simulink model "FKtest"  (Simulink 6.6)
settings: Solver=ode4  StartTime=0.0  StopTime=400  FixedStep=0.05  RelTol=1e-3
undefined symbols (not defined in the file or in its folder): amp2, vessel
libraries: marine_gnc x21, simulink x5
(part 3 of 3)

== system FKtest/Wave loads for heading2/Wave component loop/Force RAO tables/RAO interpolation in frequency5 ==
  Table : Inport
  omega : Inport  Port=2
  beta_idx : Inport  Port=3
  U_idx : Inport  Port=4
  Demux : Demux  Outputs=2
  Mux : Mux  Inputs=2
  Prelookup1 : PreLookup  BreakpointsData=vessel.forceRAO.w  BeginIndexSearchUsingPreviousIndexResult=on  ProcessOutOfRangeInput=Linear extrapolation
  Product : Product  RndMeth=Zero
  Selector1 : Selector  NumberOfDimensions=3  IndexOptions=Index vector (port),Index vector (port),Index vector (port)  Indices=[1 3],1,1  OutputSizes=1,1,1
  Sum1 : Sum  Inputs=++|
  Sum2 : Sum  Inputs=++|
  Sum3 : Sum  Inputs=-+|
  Sum4 : Sum  Inputs=++|
  one : Constant
  y : Outport
  wires:
  Prelookup1/1 -> Sum2/1
  Table/1 -> Selector1/1
  beta_idx/1 -> Selector1/3
  omega/1 -> Prelookup1/1
  U_idx/1 -> Selector1/4
  Sum4/1 -> y/1
  Sum3/1 -> Product/1
  Product/1 -> Sum4/2
  Demux/1 -> Sum4/1, Sum3/1  "y1"
  Demux/2 -> Sum3/2  "y2"
  Prelookup1/2 -> Product/2  "k"
  Selector1/1 -> Demux/1  "y"
  one/1 -> Sum1/2, Sum2/2
  Sum1/1 -> Mux/2
  Sum2/1 -> Sum1/1, Mux/1
  Mux/1 -> Selector1/2

== system FKtest/Wave loads for heading2/Wave component loop/Force RAO tables/RAO interpolation in frequency6 ==
  Table : Inport
  omega : Inport  Port=2
  beta_idx : Inport  Port=3
  U_idx : Inport  Port=4
  Demux : Demux  Outputs=2
  Mux : Mux  Inputs=2
  Prelookup1 : PreLookup  BreakpointsData=vessel.forceRAO.w  BeginIndexSearchUsingPreviousIndexResult=on  ProcessOutOfRangeInput=Linear extrapolation
  Product : Product  RndMeth=Zero
  Selector1 : Selector  NumberOfDimensions=3  IndexOptions=Index vector (port),Index vector (port),Index vector (port)  Indices=[1 3],1,1  OutputSizes=1,1,1
  Sum1 : Sum  Inputs=++|
  Sum2 : Sum  Inputs=++|
  Sum3 : Sum  Inputs=-+|
  Sum4 : Sum  Inputs=++|
  one : Constant
  y : Outport
  wires:
  Prelookup1/1 -> Sum2/1
  Table/1 -> Selector1/1
  beta_idx/1 -> Selector1/3
  omega/1 -> Prelookup1/1
  U_idx/1 -> Selector1/4
  Sum4/1 -> y/1
  Sum3/1 -> Product/1
  Product/1 -> Sum4/2
  Demux/1 -> Sum4/1, Sum3/1  "y1"
  Demux/2 -> Sum3/2  "y2"
  Prelookup1/2 -> Product/2  "k"
  Selector1/1 -> Demux/1  "y"
  one/1 -> Sum1/2, Sum2/2
  Sum1/1 -> Mux/2
  Sum2/1 -> Sum1/1, Mux/1
  Mux/1 -> Selector1/2

== system FKtest/Wave loads for heading2/Wave component loop/Force RAO tables/RAO interpolation in frequency7 ==
  Table : Inport
  omega : Inport  Port=2
  beta_idx : Inport  Port=3
  U_idx : Inport  Port=4
  Demux : Demux  Outputs=2
  Mux : Mux  Inputs=2
  Prelookup1 : PreLookup  BreakpointsData=vessel.forceRAO.w  BeginIndexSearchUsingPreviousIndexResult=on  ProcessOutOfRangeInput=Linear extrapolation
  Product : Product  RndMeth=Zero
  Selector1 : Selector  NumberOfDimensions=3  IndexOptions=Index vector (port),Index vector (port),Index vector (port)  Indices=[1 3],1,1  OutputSizes=1,1,1
  Sum1 : Sum  Inputs=++|
  Sum2 : Sum  Inputs=++|
  Sum3 : Sum  Inputs=-+|
  Sum4 : Sum  Inputs=++|
  one : Constant
  y : Outport
  wires:
  Prelookup1/1 -> Sum2/1
  Table/1 -> Selector1/1
  beta_idx/1 -> Selector1/3
  omega/1 -> Prelookup1/1
  U_idx/1 -> Selector1/4
  Sum4/1 -> y/1
  Sum3/1 -> Product/1
  Product/1 -> Sum4/2
  Demux/1 -> Sum4/1, Sum3/1  "y1"
  Demux/2 -> Sum3/2  "y2"
  Prelookup1/2 -> Product/2  "k"
  Selector1/1 -> Demux/1  "y"
  one/1 -> Sum1/2, Sum2/2
  Sum1/1 -> Mux/2
  Sum2/1 -> Sum1/1, Mux/1
  Mux/1 -> Selector1/2

== system FKtest/Wave loads for heading2/Wave component loop/Force RAO tables/RAO interpolation in frequency8 ==
  Table : Inport
  omega : Inport  Port=2
  beta_idx : Inport  Port=3
  U_idx : Inport  Port=4
  Demux : Demux  Outputs=2
  Mux : Mux  Inputs=2
  Prelookup1 : PreLookup  BreakpointsData=vessel.forceRAO.w  BeginIndexSearchUsingPreviousIndexResult=on  ProcessOutOfRangeInput=Linear extrapolation
  Product : Product  RndMeth=Zero
  Selector1 : Selector  NumberOfDimensions=3  IndexOptions=Index vector (port),Index vector (port),Index vector (port)  Indices=[1 3],1,1  OutputSizes=1,1,1
  Sum1 : Sum  Inputs=++|
  Sum2 : Sum  Inputs=++|
  Sum3 : Sum  Inputs=-+|
  Sum4 : Sum  Inputs=++|
  one : Constant
  y : Outport
  wires:
  Prelookup1/1 -> Sum2/1
  Table/1 -> Selector1/1
  beta_idx/1 -> Selector1/3
  omega/1 -> Prelookup1/1
  U_idx/1 -> Selector1/4
  Sum4/1 -> y/1
  Sum3/1 -> Product/1
  Product/1 -> Sum4/2
  Demux/1 -> Sum4/1, Sum3/1  "y1"
  Demux/2 -> Sum3/2  "y2"
  Prelookup1/2 -> Product/2  "k"
  Selector1/1 -> Demux/1  "y"
  one/1 -> Sum1/2, Sum2/2
  Sum1/1 -> Mux/2
  Sum2/1 -> Sum1/1, Mux/1
  Mux/1 -> Selector1/2

== system FKtest/Wave loads for heading2/Wave component loop/Force RAO tables/RAO interpolation in frequency9 ==
  Table : Inport
  omega : Inport  Port=2
  beta_idx : Inport  Port=3
  U_idx : Inport  Port=4
  Demux : Demux  Outputs=2
  Mux : Mux  Inputs=2
  Prelookup1 : PreLookup  BreakpointsData=vessel.forceRAO.w  BeginIndexSearchUsingPreviousIndexResult=on  ProcessOutOfRangeInput=Linear extrapolation
  Product : Product  RndMeth=Zero
  Selector1 : Selector  NumberOfDimensions=3  IndexOptions=Index vector (port),Index vector (port),Index vector (port)  Indices=[1 3],1,1  OutputSizes=1,1,1
  Sum1 : Sum  Inputs=++|
  Sum2 : Sum  Inputs=++|
  Sum3 : Sum  Inputs=-+|
  Sum4 : Sum  Inputs=++|
  one : Constant
  y : Outport
  wires:
  Prelookup1/1 -> Sum2/1
  Table/1 -> Selector1/1
  beta_idx/1 -> Selector1/3
  omega/1 -> Prelookup1/1
  U_idx/1 -> Selector1/4
  Sum4/1 -> y/1
  Sum3/1 -> Product/1
  Product/1 -> Sum4/2
  Demux/1 -> Sum4/1, Sum3/1  "y1"
  Demux/2 -> Sum3/2  "y2"
  Prelookup1/2 -> Product/2  "k"
  Selector1/1 -> Demux/1  "y"
  one/1 -> Sum1/2, Sum2/2
  Sum1/1 -> Mux/2
  Sum2/1 -> Sum1/1, Mux/1
  Mux/1 -> Selector1/2

== system FKtest/Wave loads for heading2/Wave component loop/WD RAO tables/RAO interpolation in frequency1 ==
  Table : Inport
  omega : Inport  Port=2
  beta_idx : Inport  Port=3
  U_idx : Inport  Port=4
  Demux : Demux  Outputs=2
  Mux : Mux  Inputs=2
  Prelookup1 : PreLookup  BreakpointsData=vessel.forceRAO.w  BeginIndexSearchUsingPreviousIndexResult=on  ProcessOutOfRangeInput=Linear extrapolation
  Product : Product  RndMeth=Zero
  Selector1 : Selector  NumberOfDimensions=3  IndexOptions=Index vector (port),Index vector (port),Index vector (port)  Indices=[1 3],1,1  OutputSizes=1,1,1
  Sum1 : Sum  Inputs=++|
  Sum2 : Sum  Inputs=++|
  Sum3 : Sum  Inputs=-+|
  Sum4 : Sum  Inputs=++|
  one : Constant
  y : Outport
  wires:
  Prelookup1/1 -> Sum2/1
  Table/1 -> Selector1/1
  beta_idx/1 -> Selector1/3
  omega/1 -> Prelookup1/1
  U_idx/1 -> Selector1/4
  Sum4/1 -> y/1
  Sum3/1 -> Product/1
  Product/1 -> Sum4/2
  Demux/1 -> Sum4/1, Sum3/1  "y1"
  Demux/2 -> Sum3/2  "y2"
  Prelookup1/2 -> Product/2  "k"
  Selector1/1 -> Demux/1  "y"
  one/1 -> Sum1/2, Sum2/2
  Sum1/1 -> Mux/2
  Sum2/1 -> Sum1/1, Mux/1
  Mux/1 -> Selector1/2

== system FKtest/Wave loads for heading2/Wave component loop/WD RAO tables/RAO interpolation in frequency2 ==
  Table : Inport
  omega : Inport  Port=2
  beta_idx : Inport  Port=3
  U_idx : Inport  Port=4
  Demux : Demux  Outputs=2
  Mux : Mux  Inputs=2
  Prelookup1 : PreLookup  BreakpointsData=vessel.forceRAO.w  BeginIndexSearchUsingPreviousIndexResult=on  ProcessOutOfRangeInput=Linear extrapolation
  Product : Product  RndMeth=Zero
  Selector1 : Selector  NumberOfDimensions=3  IndexOptions=Index vector (port),Index vector (port),Index vector (port)  Indices=[1 3],1,1  OutputSizes=1,1,1
  Sum1 : Sum  Inputs=++|
  Sum2 : Sum  Inputs=++|
  Sum3 : Sum  Inputs=-+|
  Sum4 : Sum  Inputs=++|
  one : Constant
  y : Outport
  wires:
  Prelookup1/1 -> Sum2/1
  Table/1 -> Selector1/1
  beta_idx/1 -> Selector1/3
  omega/1 -> Prelookup1/1
  U_idx/1 -> Selector1/4
  Sum4/1 -> y/1
  Sum3/1 -> Product/1
  Product/1 -> Sum4/2
  Demux/1 -> Sum4/1, Sum3/1  "y1"
  Demux/2 -> Sum3/2  "y2"
  Prelookup1/2 -> Product/2  "k"
  Selector1/1 -> Demux/1  "y"
  one/1 -> Sum1/2, Sum2/2
  Sum1/1 -> Mux/2
  Sum2/1 -> Sum1/1, Mux/1
  Mux/1 -> Selector1/2

== system FKtest/Wave loads for heading2/Wave component loop/WD RAO tables/RAO interpolation in frequency3 ==
  Table : Inport
  omega : Inport  Port=2
  beta_idx : Inport  Port=3
  U_idx : Inport  Port=4
  Demux : Demux  Outputs=2
  Mux : Mux  Inputs=2
  Prelookup1 : PreLookup  BreakpointsData=vessel.forceRAO.w  BeginIndexSearchUsingPreviousIndexResult=on  ProcessOutOfRangeInput=Linear extrapolation
  Product : Product  RndMeth=Zero
  Selector1 : Selector  NumberOfDimensions=3  IndexOptions=Index vector (port),Index vector (port),Index vector (port)  Indices=[1 3],1,1  OutputSizes=1,1,1
  Sum1 : Sum  Inputs=++|
  Sum2 : Sum  Inputs=++|
  Sum3 : Sum  Inputs=-+|
  Sum4 : Sum  Inputs=++|
  one : Constant
  y : Outport
  wires:
  Prelookup1/1 -> Sum2/1
  Table/1 -> Selector1/1
  beta_idx/1 -> Selector1/3
  omega/1 -> Prelookup1/1
  U_idx/1 -> Selector1/4
  Sum4/1 -> y/1
  Sum3/1 -> Product/1
  Product/1 -> Sum4/2
  Demux/1 -> Sum4/1, Sum3/1  "y1"
  Demux/2 -> Sum3/2  "y2"
  Prelookup1/2 -> Product/2  "k"
  Selector1/1 -> Demux/1  "y"
  one/1 -> Sum1/2, Sum2/2
  Sum1/1 -> Mux/2
  Sum2/1 -> Sum1/1, Mux/1
  Mux/1 -> Selector1/2
